simulink model "ModelG"  (Simulink 7.4)
settings: Solver=ode45  StartTime=0.0  StopTime=400  RelTol=1e-5
undefined symbols (not defined in the file): magnitude
settings Model: Creator=Lluís  LastModifiedBy=Lluís

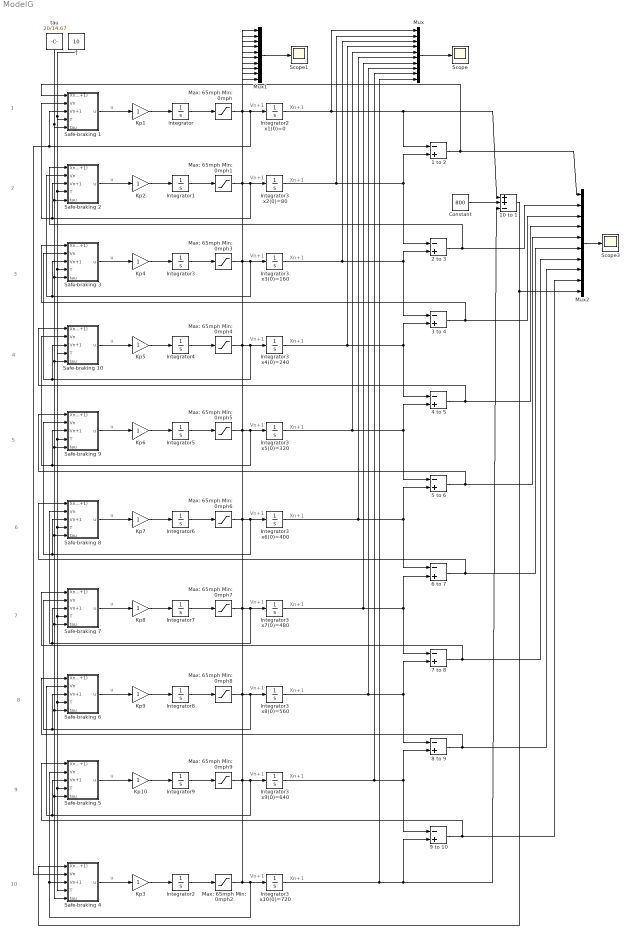
== system ModelG ==
  note: u
  note: Vn+1
  note: Xn+1
  note: u
  note: Vn+1
  note: Xn+1
  note: 1
  note: 2
  note: u
  note: Vn+1
  note: Xn+1
  note: 10
  note: u
  note: Vn+1
  note: Xn+1
  note: 3
  note: u
  note: Vn+1
  note: Xn+1
  note: 4
  note: u
  note: Vn+1
  note: Xn+1
  note: 5
  note: u
  note: Vn+1
  note: Xn+1
  note: 6
  note: u
  note: Vn+1
  note: Xn+1
  note: 7
  note: u
  note: Vn+1
  note: Xn+1
  note: 8
  note: u
  note: Vn+1
  note: Xn+1
  note: 9
  1 to 2 : Sum  Inputs=-+  OutDataType=fixdt(1, 16)  OutScaling=2^-10
  10 to 1 : Sum  Inputs=++-  OutDataType=fixdt(1, 16)  OutScaling=2^-10
  2 to 3 : Sum  Inputs=-+  OutDataType=fixdt(1, 16)  OutScaling=2^-10
  3 to 4 : Sum  Inputs=-+  OutDataType=fixdt(1, 16)  OutScaling=2^-10
  4 to 5 : Sum  Inputs=-+  OutDataType=fixdt(1, 16)  OutScaling=2^-10
  5 to 6 : Sum  Inputs=-+  OutDataType=fixdt(1, 16)  OutScaling=2^-10
  6 to 7 : Sum  Inputs=-+  OutDataType=fixdt(1, 16)  OutScaling=2^-10
  7 to 8 : Sum  Inputs=-+  OutDataType=fixdt(1, 16)  OutScaling=2^-10
  8 to 9 : Sum  Inputs=-+  OutDataType=fixdt(1, 16)  OutScaling=2^-10
  9 to 10 : Sum  Inputs=-+  OutDataType=fixdt(1, 16)  OutScaling=2^-10
  Constant : Constant  Value=800  OutDataType=fixdt(1, 16)  OutScaling=2^0
  Integrator : Integrator  InitialCondition=22
  Integrator{1..2,4,6,8} (5 alike) : Integrator  InitialCondition=66
  Integrator2 x1(0)=0 : Integrator
  Integrator3 : Integrator  InitialCondition=44
  Integrator3 x10(0)=720 : Integrator  InitialCondition=720
  Integrator3 x2(0)=80 : Integrator  InitialCondition=80
  Integrator3 x3(0)=160 : Integrator  InitialCondition=160
  Integrator3 x4(0)=240 : Integrator  InitialCondition=240
  Integrator3 x5(0)=320 : Integrator  InitialCondition=320
  Integrator3 x6(0)=400 : Integrator  InitialCondition=400
  Integrator3 x7(0)=480 : Integrator  InitialCondition=480
  Integrator3 x8(0)=560 : Integrator  InitialCondition=560
  Integrator3 x9(0)=640 : Integrator  InitialCondition=640
  Integrator5 : Integrator  InitialCondition=22
  Integrator7 : Integrator  InitialCondition=44
  Integrator9 : Integrator  InitialCondition=22
  Kp{1..10} (10 alike) : Gain  ParameterDataType=fixdt(1, 16)  ParameterScaling=2^0  OutDataType=fixdt(1, 16)  OutScaling=2^0
  Max: 65mph Min: 0mph{,1..9} (10 alike) : Saturate  UpperLimit=95.33  LowerLimit=0  OutDataType=fixdt(1, 16)  OutScaling=2^0
  Mux : Mux  Inputs=10
  Mux1 : Mux  Inputs=10
  Mux2 : Mux  Inputs=10
  Safe-braking 1 : Subsystem
  Safe-braking 10 : Subsystem
  Safe-braking 2 : Subsystem
  Safe-braking 3 : Subsystem
  Safe-braking 4 : Subsystem
  Safe-braking 5 : Subsystem
  Safe-braking 6 : Subsystem
  Safe-braking 7 : Subsystem
  Safe-braking 8 : Subsystem
  Safe-braking 9 : Subsystem
  Scope : Scope
      settings: SaveName=pos  DataFormat=Array
  Scope1 : Scope
      settings: SaveName=speed
  Scope3 : Scope
      settings: SaveName=ScopeData3
  T : Constant  Value=10  OutDataType=fixdt(1, 16)  OutScaling=2^0
  tau : Constant  Value=20/14.67  OutDataType=fixdt(1, 16)  OutScaling=2^0
  wires:
  1 to 2/1 -> Safe-braking 1/1(Xn-(Xn+1)), Mux2/1
  Max: 65mph Min: 0mph/1 -> Integrator2 x1(0)=0/1, Safe-braking 1/3(Vn+1), Safe-braking 4/2(Vn), Mux1/1
  Kp1/1 -> Integrator/1
  Safe-braking 1/1(u) -> Kp1/1
  Integrator/1 -> Max: 65mph Min: 0mph/1
  Integrator2 x1(0)=0/1 -> 1 to 2/1, 10 to 1/1, Mux/1
  Max: 65mph Min: 0mph1/1 -> Safe-braking 1/2(Vn), Safe-braking 2/3(Vn+1), Integrator3 x2(0)=80/1, Mux1/2
  Kp2/1 -> Integrator1/1
  Safe-braking 2/1(u) -> Kp2/1
  Integrator1/1 -> Max: 65mph Min: 0mph1/1
  Integrator3 x2(0)=80/1 -> 1 to 2/2, 2 to 3/1, Mux/2
  Max: 65mph Min: 0mph2/1 -> Integrator3 x10(0)=720/1, Safe-braking 4/3(Vn+1), Safe-braking 5/2(Vn), Mux1/10
  Kp3/1 -> Integrator2/1
  Safe-braking 4/1(u) -> Kp3/1
  Integrator2/1 -> Max: 65mph Min: 0mph2/1
  Integrator3 x10(0)=720/1 -> 10 to 1/3, 9 to 10/2, Mux/10
  2 to 3/1 -> Mux2/2, Safe-braking 2/1(Xn-(Xn+1))
  Constant/1 -> 10 to 1/2
  10 to 1/1 -> Mux2/10, Safe-braking 4/1(Xn-(Xn+1))
  Mux/1 -> Scope/1
  Mux1/1 -> Scope1/1
  Mux2/1 -> Scope3/1
  Max: 65mph Min: 0mph3/1 -> Integrator3 x3(0)=160/1, Safe-braking 2/2(Vn), Safe-braking 3/3(Vn+1), Mux1/3
  Kp4/1 -> Integrator3/1
  Safe-braking 3/1(u) -> Kp4/1
  Integrator3/1 -> Max: 65mph Min: 0mph3/1
  Integrator3 x3(0)=160/1 -> 2 to 3/2, 3 to 4/1, Mux/3
  3 to 4/1 -> Mux2/3, Safe-braking 3/1(Xn-(Xn+1))
  Max: 65mph Min: 0mph4/1 -> Integrator3 x4(0)=240/1, Safe-braking 3/2(Vn), Safe-braking 10/3(Vn+1), Mux1/4
  Kp5/1 -> Integrator4/1
  Safe-braking 10/1(u) -> Kp5/1
  Integrator4/1 -> Max: 65mph Min: 0mph4/1
  Integrator3 x4(0)=240/1 -> 3 to 4/2, 4 to 5/1, Mux/4
  4 to 5/1 -> Mux2/4, Safe-braking 10/1(Xn-(Xn+1))
  Max: 65mph Min: 0mph5/1 -> Integrator3 x5(0)=320/1, Safe-braking 9/3(Vn+1), Safe-braking 10/2(Vn), Mux1/5
  Kp6/1 -> Integrator5/1
  Safe-braking 9/1(u) -> Kp6/1
  Integrator5/1 -> Max: 65mph Min: 0mph5/1
  Integrator3 x5(0)=320/1 -> 4 to 5/2, 5 to 6/1, Mux/5
  5 to 6/1 -> Mux2/5, Safe-braking 9/1(Xn-(Xn+1))
  Max: 65mph Min: 0mph6/1 -> Integrator3 x6(0)=400/1, Safe-braking 8/3(Vn+1), Safe-braking 9/2(Vn), Mux1/6
  Kp7/1 -> Integrator6/1
  Safe-braking 8/1(u) -> Kp7/1
  Integrator6/1 -> Max: 65mph Min: 0mph6/1
  Integrator3 x6(0)=400/1 -> 5 to 6/2, 6 to 7/1, Mux/6
  6 to 7/1 -> Mux2/6, Safe-braking 8/1(Xn-(Xn+1))
  Max: 65mph Min: 0mph7/1 -> Integrator3 x7(0)=480/1, Safe-braking 7/3(Vn+1), Safe-braking 8/2(Vn), Mux1/7
  Kp8/1 -> Integrator7/1
  Safe-braking 7/1(u) -> Kp8/1
  Integrator7/1 -> Max: 65mph Min: 0mph7/1
  Integrator3 x7(0)=480/1 -> 6 to 7/2, 7 to 8/1, Mux/7
  7 to 8/1 -> Mux2/7, Safe-braking 7/1(Xn-(Xn+1))
  Max: 65mph Min: 0mph8/1 -> Integrator3 x8(0)=560/1, Safe-braking 6/3(Vn+1), Safe-braking 7/2(Vn), Mux1/8
  Kp9/1 -> Integrator8/1
  Safe-braking 6/1(u) -> Kp9/1
  Integrator8/1 -> Max: 65mph Min: 0mph8/1
  Integrator3 x8(0)=560/1 -> 7 to 8/2, 8 to 9/1, Mux/8
  8 to 9/1 -> Mux2/8, Safe-braking 6/1(Xn-(Xn+1))
  Max: 65mph Min: 0mph9/1 -> Integrator3 x9(0)=640/1, Safe-braking 5/3(Vn+1), Safe-braking 6/2(Vn), Mux1/9
  Kp10/1 -> Integrator9/1
  Safe-braking 5/1(u) -> Kp10/1
  Integrator9/1 -> Max: 65mph Min: 0mph9/1
  Integrator3 x9(0)=640/1 -> 8 to 9/2, 9 to 10/1, Mux/9
  9 to 10/1 -> Mux2/9, Safe-braking 5/1(Xn-(Xn+1))
  T/1 -> Safe-braking 2/4(T), Safe-braking 3/4(T), Safe-braking 9/4(T), Safe-braking 8/4(T), Safe-braking 7/4(T), Safe-braking 6/4(T), Safe-braking 5/4(T), Safe-braking 4/4(T), Safe-braking 10/4(T), Safe-braking 1/4(T)
  tau/1 -> Safe-braking 2/5(tau), Safe-braking 3/5(tau), Safe-braking 10/5(tau), Safe-braking 9/5(tau), Safe-braking 8/5(tau), Safe-braking 7/5(tau), Safe-braking 6/5(tau), Safe-braking 5/5(tau), Safe-braking 4/5(tau), Safe-braking 1/5(tau)

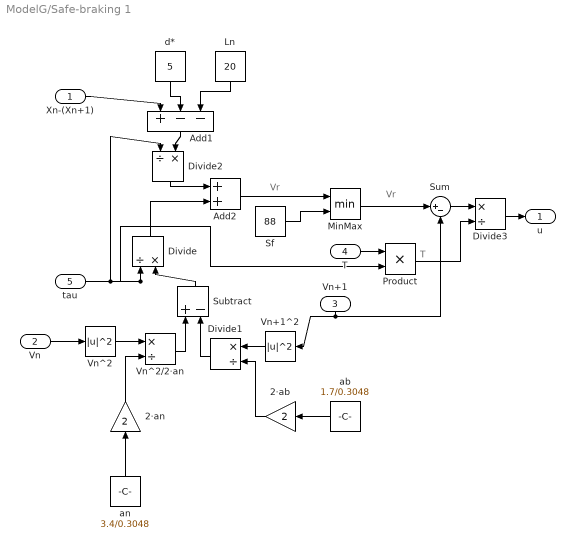
== system ModelG/Safe-braking 1 ==
  note: Vr
  note: Vr
  note: T
  Xn-(Xn+1) : Inport
  Vn : Inport  Port=2
  Vn+1 : Inport  Port=3
  T : Inport  Port=4  OutDataType=fixdt(1, 16)  OutScaling=2^0
  tau : Inport  Port=5  OutDataType=fixdt(1, 16)  OutScaling=2^0
  2·ab : Gain  Gain=2  ParameterDataType=fixdt(1, 16)  ParameterScaling=2^0  OutDataType=fixdt(1, 16)  OutScaling=2^0
  2·an : Gain  Gain=2  ParameterDataType=fixdt(1, 16)  ParameterScaling=2^0  OutDataType=fixdt(1, 16)  OutScaling=2^0
  Add1 : Sum  Inputs=+--  OutDataType=fixdt(1, 16)  OutScaling=2^-10
  Add2 : Sum  OutDataType=fixdt(1, 16)  OutScaling=2^-10
  Divide : Product  Inputs=/*  OutDataType=fixdt(1, 16)  OutScaling=2^-10
  Divide1 : Product  Inputs=*/  OutDataType=fixdt(1, 16)  OutScaling=2^-10
  Divide2 : Product  Inputs=/*  OutDataType=fixdt(1, 16)  OutScaling=2^-10
  Divide3 : Product  Inputs=*/  OutDataType=fixdt(1, 16)  OutScaling=2^-10
  Ln : Constant  Value=20  OutDataType=fixdt(1, 16)  OutScaling=2^0
  MinMax : MinMax  Inputs=2  OutDataType=fixdt(1, 16)  OutScaling=2^0
  Product : Product  OutDataType=fixdt(1, 16)  OutScaling=2^0  RndMeth=Zero
  Sf : Constant  Value=88  OutDataType=fixdt(1, 16)  OutScaling=2^0
  Subtract : Sum  Inputs=+-  OutDataType=fixdt(1, 16)  OutScaling=2^-10
  Sum : Sum  Inputs=|+-  OutDataType=fixdt(1, 16)  OutScaling=2^0
  Vn+1^2 : Math  Operator=magnitude^2  OutDataType=fixdt(1, 16)  OutScaling=2^0  SaturateOnIntegerOverflow=on
  Vn^2 : Math  Operator=magnitude^2  OutDataType=fixdt(1, 16)  OutScaling=2^0  SaturateOnIntegerOverflow=on
  Vn^2/2·an : Product  Inputs=*/  OutDataType=fixdt(1, 16)  OutScaling=2^-10
  ab : Constant  Value=1.7/0.3048  OutDataType=fixdt(1, 16)  OutScaling=2^0
  an : Constant  Value=3.4/0.3048  OutDataType=fixdt(1, 16)  OutScaling=2^0
  d* : Constant  Value=5  OutDataType=fixdt(1, 16)  OutScaling=2^0
  u : Outport
  wires:
  ab/1 -> 2·ab/1
  Vn^2/1 -> Vn^2/2·an/1
  2·an/1 -> Vn^2/2·an/2
  Vn+1^2/1 -> Divide1/1
  2·ab/1 -> Divide1/2
  Vn^2/2·an/1 -> Subtract/1
  Divide1/1 -> Subtract/2
  Subtract/1 -> Divide/2
  tau/1 -> Divide2/1, Divide/1, Product/2
  d*/1 -> Add1/2
  Ln/1 -> Add1/3
  Add1/1 -> Divide2/2
  Divide2/1 -> Add2/1
  Divide/1 -> Add2/2
  Xn-(Xn+1)/1 -> Add1/1
  Vn/1 -> Vn^2/1
  Vn+1/1 -> Vn+1^2/1, Sum/2
  an/1 -> 2·an/1
  Add2/1 -> MinMax/1
  Sf/1 -> MinMax/2
  MinMax/1 -> Sum/1
  Sum/1 -> Divide3/1
  Product/1 -> Divide3/2
  Divide3/1 -> u/1
  T/1 -> Product/1

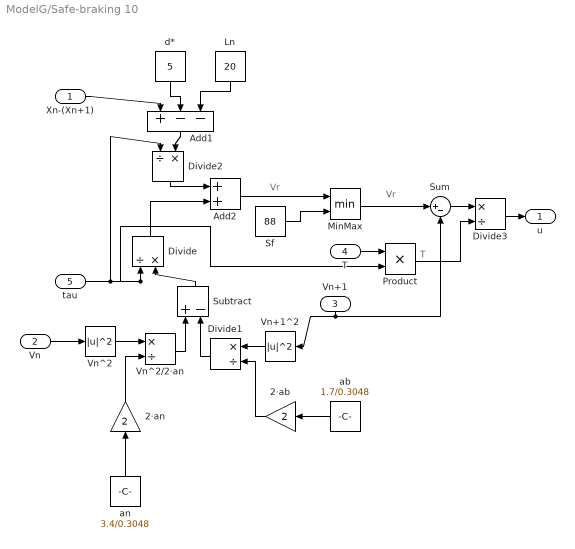
== system ModelG/Safe-braking 10 ==
  note: Vr
  note: Vr
  note: T
  Xn-(Xn+1) : Inport
  Vn : Inport  Port=2
  Vn+1 : Inport  Port=3
  T : Inport  Port=4  OutDataType=fixdt(1, 16)  OutScaling=2^0
  tau : Inport  Port=5  OutDataType=fixdt(1, 16)  OutScaling=2^0
  2·ab : Gain  Gain=2  ParameterDataType=fixdt(1, 16)  ParameterScaling=2^0  OutDataType=fixdt(1, 16)  OutScaling=2^0
  2·an : Gain  Gain=2  ParameterDataType=fixdt(1, 16)  ParameterScaling=2^0  OutDataType=fixdt(1, 16)  OutScaling=2^0
  Add1 : Sum  Inputs=+--  OutDataType=fixdt(1, 16)  OutScaling=2^-10
  Add2 : Sum  OutDataType=fixdt(1, 16)  OutScaling=2^-10
  Divide : Product  Inputs=/*  OutDataType=fixdt(1, 16)  OutScaling=2^-10
  Divide1 : Product  Inputs=*/  OutDataType=fixdt(1, 16)  OutScaling=2^-10
  Divide2 : Product  Inputs=/*  OutDataType=fixdt(1, 16)  OutScaling=2^-10
  Divide3 : Product  Inputs=*/  OutDataType=fixdt(1, 16)  OutScaling=2^-10
  Ln : Constant  Value=20  OutDataType=fixdt(1, 16)  OutScaling=2^0
  MinMax : MinMax  Inputs=2  OutDataType=fixdt(1, 16)  OutScaling=2^0
  Product : Product  OutDataType=fixdt(1, 16)  OutScaling=2^0  RndMeth=Zero
  Sf : Constant  Value=88  OutDataType=fixdt(1, 16)  OutScaling=2^0
  Subtract : Sum  Inputs=+-  OutDataType=fixdt(1, 16)  OutScaling=2^-10
  Sum : Sum  Inputs=|+-  OutDataType=fixdt(1, 16)  OutScaling=2^0
  Vn+1^2 : Math  Operator=magnitude^2  OutDataType=fixdt(1, 16)  OutScaling=2^0  SaturateOnIntegerOverflow=on
  Vn^2 : Math  Operator=magnitude^2  OutDataType=fixdt(1, 16)  OutScaling=2^0  SaturateOnIntegerOverflow=on
  Vn^2/2·an : Product  Inputs=*/  OutDataType=fixdt(1, 16)  OutScaling=2^-10
  ab : Constant  Value=1.7/0.3048  OutDataType=fixdt(1, 16)  OutScaling=2^0
  an : Constant  Value=3.4/0.3048  OutDataType=fixdt(1, 16)  OutScaling=2^0
  d* : Constant  Value=5  OutDataType=fixdt(1, 16)  OutScaling=2^0
  u : Outport
  wires:
  ab/1 -> 2·ab/1
  Vn^2/1 -> Vn^2/2·an/1
  2·an/1 -> Vn^2/2·an/2
  Vn+1^2/1 -> Divide1/1
  2·ab/1 -> Divide1/2
  Vn^2/2·an/1 -> Subtract/1
  Divide1/1 -> Subtract/2
  Subtract/1 -> Divide/2
  tau/1 -> Divide2/1, Divide/1, Product/2
  d*/1 -> Add1/2
  Ln/1 -> Add1/3
  Add1/1 -> Divide2/2
  Divide2/1 -> Add2/1
  Divide/1 -> Add2/2
  Xn-(Xn+1)/1 -> Add1/1
  Vn/1 -> Vn^2/1
  Vn+1/1 -> Vn+1^2/1, Sum/2
  an/1 -> 2·an/1
  Add2/1 -> MinMax/1
  Sf/1 -> MinMax/2
  MinMax/1 -> Sum/1
  Sum/1 -> Divide3/1
  Product/1 -> Divide3/2
  Divide3/1 -> u/1
  T/1 -> Product/1

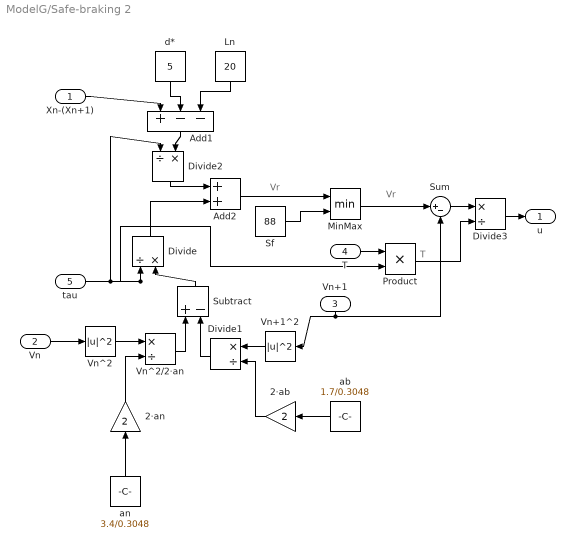
== system ModelG/Safe-braking 2 ==
  note: Vr
  note: Vr
  note: T
  Xn-(Xn+1) : Inport
  Vn : Inport  Port=2
  Vn+1 : Inport  Port=3
  T : Inport  Port=4  OutDataType=fixdt(1, 16)  OutScaling=2^0
  tau : Inport  Port=5  OutDataType=fixdt(1, 16)  OutScaling=2^0
  2·ab : Gain  Gain=2  ParameterDataType=fixdt(1, 16)  ParameterScaling=2^0  OutDataType=fixdt(1, 16)  OutScaling=2^0
  2·an : Gain  Gain=2  ParameterDataType=fixdt(1, 16)  ParameterScaling=2^0  OutDataType=fixdt(1, 16)  OutScaling=2^0
  Add1 : Sum  Inputs=+--  OutDataType=fixdt(1, 16)  OutScaling=2^-10
  Add2 : Sum  OutDataType=fixdt(1, 16)  OutScaling=2^-10
  Divide : Product  Inputs=/*  OutDataType=fixdt(1, 16)  OutScaling=2^-10
  Divide1 : Product  Inputs=*/  OutDataType=fixdt(1, 16)  OutScaling=2^-10
  Divide2 : Product  Inputs=/*  OutDataType=fixdt(1, 16)  OutScaling=2^-10
  Divide3 : Product  Inputs=*/  OutDataType=fixdt(1, 16)  OutScaling=2^-10
  Ln : Constant  Value=20  OutDataType=fixdt(1, 16)  OutScaling=2^0
  MinMax : MinMax  Inputs=2  OutDataType=fixdt(1, 16)  OutScaling=2^0
  Product : Product  OutDataType=fixdt(1, 16)  OutScaling=2^0  RndMeth=Zero
  Sf : Constant  Value=88  OutDataType=fixdt(1, 16)  OutScaling=2^0
  Subtract : Sum  Inputs=+-  OutDataType=fixdt(1, 16)  OutScaling=2^-10
  Sum : Sum  Inputs=|+-  OutDataType=fixdt(1, 16)  OutScaling=2^0
  Vn+1^2 : Math  Operator=magnitude^2  OutDataType=fixdt(1, 16)  OutScaling=2^0  SaturateOnIntegerOverflow=on
  Vn^2 : Math  Operator=magnitude^2  OutDataType=fixdt(1, 16)  OutScaling=2^0  SaturateOnIntegerOverflow=on
  Vn^2/2·an : Product  Inputs=*/  OutDataType=fixdt(1, 16)  OutScaling=2^-10
  ab : Constant  Value=1.7/0.3048  OutDataType=fixdt(1, 16)  OutScaling=2^0
  an : Constant  Value=3.4/0.3048  OutDataType=fixdt(1, 16)  OutScaling=2^0
  d* : Constant  Value=5  OutDataType=fixdt(1, 16)  OutScaling=2^0
  u : Outport
  wires:
  ab/1 -> 2·ab/1
  Vn^2/1 -> Vn^2/2·an/1
  2·an/1 -> Vn^2/2·an/2
  Vn+1^2/1 -> Divide1/1
  2·ab/1 -> Divide1/2
  Vn^2/2·an/1 -> Subtract/1
  Divide1/1 -> Subtract/2
  Subtract/1 -> Divide/2
  tau/1 -> Divide2/1, Divide/1, Product/2
  d*/1 -> Add1/2
  Ln/1 -> Add1/3
  Add1/1 -> Divide2/2
  Divide2/1 -> Add2/1
  Divide/1 -> Add2/2
  Xn-(Xn+1)/1 -> Add1/1
  Vn/1 -> Vn^2/1
  Vn+1/1 -> Vn+1^2/1, Sum/2
  an/1 -> 2·an/1
  Add2/1 -> MinMax/1
  Sf/1 -> MinMax/2
  MinMax/1 -> Sum/1
  Sum/1 -> Divide3/1
  Product/1 -> Divide3/2
  Divide3/1 -> u/1
  T/1 -> Product/1

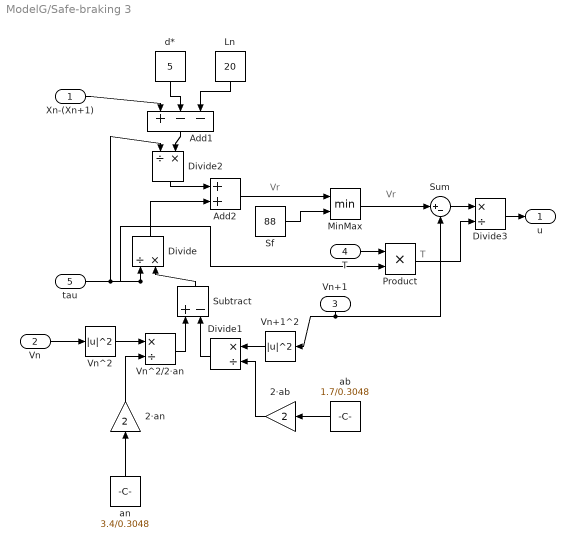
== system ModelG/Safe-braking 3 ==
  note: Vr
  note: Vr
  note: T
  Xn-(Xn+1) : Inport
  Vn : Inport  Port=2
  Vn+1 : Inport  Port=3
  T : Inport  Port=4  OutDataType=fixdt(1, 16)  OutScaling=2^0
  tau : Inport  Port=5  OutDataType=fixdt(1, 16)  OutScaling=2^0
  2·ab : Gain  Gain=2  ParameterDataType=fixdt(1, 16)  ParameterScaling=2^0  OutDataType=fixdt(1, 16)  OutScaling=2^0
  2·an : Gain  Gain=2  ParameterDataType=fixdt(1, 16)  ParameterScaling=2^0  OutDataType=fixdt(1, 16)  OutScaling=2^0
  Add1 : Sum  Inputs=+--  OutDataType=fixdt(1, 16)  OutScaling=2^-10
  Add2 : Sum  OutDataType=fixdt(1, 16)  OutScaling=2^-10
  Divide : Product  Inputs=/*  OutDataType=fixdt(1, 16)  OutScaling=2^-10
  Divide1 : Product  Inputs=*/  OutDataType=fixdt(1, 16)  OutScaling=2^-10
  Divide2 : Product  Inputs=/*  OutDataType=fixdt(1, 16)  OutScaling=2^-10
  Divide3 : Product  Inputs=*/  OutDataType=fixdt(1, 16)  OutScaling=2^-10
  Ln : Constant  Value=20  OutDataType=fixdt(1, 16)  OutScaling=2^0
  MinMax : MinMax  Inputs=2  OutDataType=fixdt(1, 16)  OutScaling=2^0
  Product : Product  OutDataType=fixdt(1, 16)  OutScaling=2^0  RndMeth=Zero
  Sf : Constant  Value=88  OutDataType=fixdt(1, 16)  OutScaling=2^0
  Subtract : Sum  Inputs=+-  OutDataType=fixdt(1, 16)  OutScaling=2^-10
  Sum : Sum  Inputs=|+-  OutDataType=fixdt(1, 16)  OutScaling=2^0
  Vn+1^2 : Math  Operator=magnitude^2  OutDataType=fixdt(1, 16)  OutScaling=2^0  SaturateOnIntegerOverflow=on
  Vn^2 : Math  Operator=magnitude^2  OutDataType=fixdt(1, 16)  OutScaling=2^0  SaturateOnIntegerOverflow=on
  Vn^2/2·an : Product  Inputs=*/  OutDataType=fixdt(1, 16)  OutScaling=2^-10
  ab : Constant  Value=1.7/0.3048  OutDataType=fixdt(1, 16)  OutScaling=2^0
  an : Constant  Value=3.4/0.3048  OutDataType=fixdt(1, 16)  OutScaling=2^0
  d* : Constant  Value=5  OutDataType=fixdt(1, 16)  OutScaling=2^0
  u : Outport
  wires:
  ab/1 -> 2·ab/1
  Vn^2/1 -> Vn^2/2·an/1
  2·an/1 -> Vn^2/2·an/2
  Vn+1^2/1 -> Divide1/1
  2·ab/1 -> Divide1/2
  Vn^2/2·an/1 -> Subtract/1
  Divide1/1 -> Subtract/2
  Subtract/1 -> Divide/2
  tau/1 -> Divide2/1, Divide/1, Product/2
  d*/1 -> Add1/2
  Ln/1 -> Add1/3
  Add1/1 -> Divide2/2
  Divide2/1 -> Add2/1
  Divide/1 -> Add2/2
  Xn-(Xn+1)/1 -> Add1/1
  Vn/1 -> Vn^2/1
  Vn+1/1 -> Vn+1^2/1, Sum/2
  an/1 -> 2·an/1
  Add2/1 -> MinMax/1
  Sf/1 -> MinMax/2
  MinMax/1 -> Sum/1
  Sum/1 -> Divide3/1
  Product/1 -> Divide3/2
  Divide3/1 -> u/1
  T/1 -> Product/1

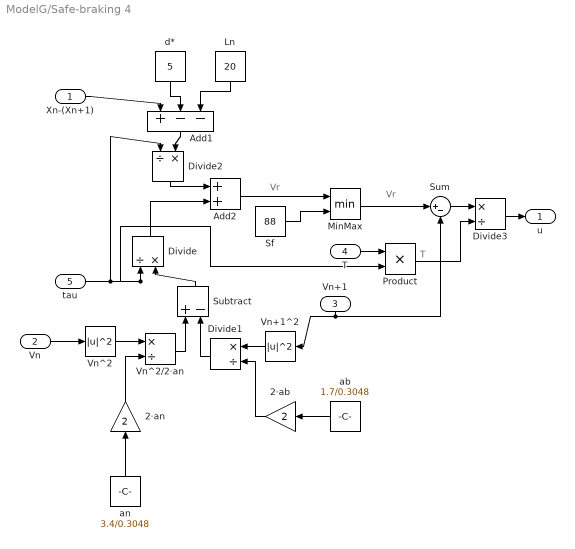
== system ModelG/Safe-braking 4 ==
  note: Vr
  note: Vr
  note: T
  Xn-(Xn+1) : Inport
  Vn : Inport  Port=2
  Vn+1 : Inport  Port=3
  T : Inport  Port=4  OutDataType=fixdt(1, 16)  OutScaling=2^0
  tau : Inport  Port=5  OutDataType=fixdt(1, 16)  OutScaling=2^0
  2·ab : Gain  Gain=2  ParameterDataType=fixdt(1, 16)  ParameterScaling=2^0  OutDataType=fixdt(1, 16)  OutScaling=2^0
  2·an : Gain  Gain=2  ParameterDataType=fixdt(1, 16)  ParameterScaling=2^0  OutDataType=fixdt(1, 16)  OutScaling=2^0
  Add1 : Sum  Inputs=+--  OutDataType=fixdt(1, 16)  OutScaling=2^-10
  Add2 : Sum  OutDataType=fixdt(1, 16)  OutScaling=2^-10
  Divide : Product  Inputs=/*  OutDataType=fixdt(1, 16)  OutScaling=2^-10
  Divide1 : Product  Inputs=*/  OutDataType=fixdt(1, 16)  OutScaling=2^-10
  Divide2 : Product  Inputs=/*  OutDataType=fixdt(1, 16)  OutScaling=2^-10
  Divide3 : Product  Inputs=*/  OutDataType=fixdt(1, 16)  OutScaling=2^-10
  Ln : Constant  Value=20  OutDataType=fixdt(1, 16)  OutScaling=2^0
  MinMax : MinMax  Inputs=2  OutDataType=fixdt(1, 16)  OutScaling=2^0
  Product : Product  OutDataType=fixdt(1, 16)  OutScaling=2^0  RndMeth=Zero
  Sf : Constant  Value=88  OutDataType=fixdt(1, 16)  OutScaling=2^0
  Subtract : Sum  Inputs=+-  OutDataType=fixdt(1, 16)  OutScaling=2^-10
  Sum : Sum  Inputs=|+-  OutDataType=fixdt(1, 16)  OutScaling=2^0
  Vn+1^2 : Math  Operator=magnitude^2  OutDataType=fixdt(1, 16)  OutScaling=2^0  SaturateOnIntegerOverflow=on
  Vn^2 : Math  Operator=magnitude^2  OutDataType=fixdt(1, 16)  OutScaling=2^0  SaturateOnIntegerOverflow=on
  Vn^2/2·an : Product  Inputs=*/  OutDataType=fixdt(1, 16)  OutScaling=2^-10
  ab : Constant  Value=1.7/0.3048  OutDataType=fixdt(1, 16)  OutScaling=2^0
  an : Constant  Value=3.4/0.3048  OutDataType=fixdt(1, 16)  OutScaling=2^0
  d* : Constant  Value=5  OutDataType=fixdt(1, 16)  OutScaling=2^0
  u : Outport
  wires:
  ab/1 -> 2·ab/1
  Vn^2/1 -> Vn^2/2·an/1
  2·an/1 -> Vn^2/2·an/2
  Vn+1^2/1 -> Divide1/1
  2·ab/1 -> Divide1/2
  Vn^2/2·an/1 -> Subtract/1
  Divide1/1 -> Subtract/2
  Subtract/1 -> Divide/2
  tau/1 -> Divide2/1, Divide/1, Product/2
  d*/1 -> Add1/2
  Ln/1 -> Add1/3
  Add1/1 -> Divide2/2
  Divide2/1 -> Add2/1
  Divide/1 -> Add2/2
  Xn-(Xn+1)/1 -> Add1/1
  Vn/1 -> Vn^2/1
  Vn+1/1 -> Vn+1^2/1, Sum/2
  an/1 -> 2·an/1
  Add2/1 -> MinMax/1
  Sf/1 -> MinMax/2
  MinMax/1 -> Sum/1
  Sum/1 -> Divide3/1
  Product/1 -> Divide3/2
  Divide3/1 -> u/1
  T/1 -> Product/1

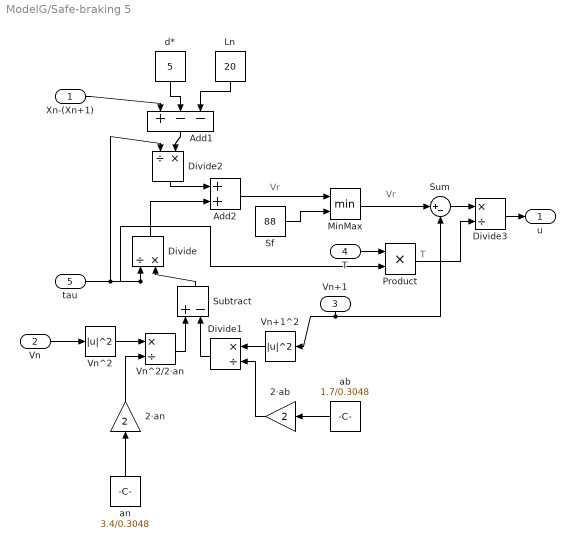
== system ModelG/Safe-braking 5 ==
  note: Vr
  note: Vr
  note: T
  Xn-(Xn+1) : Inport
  Vn : Inport  Port=2
  Vn+1 : Inport  Port=3
  T : Inport  Port=4  OutDataType=fixdt(1, 16)  OutScaling=2^0
  tau : Inport  Port=5  OutDataType=fixdt(1, 16)  OutScaling=2^0
  2·ab : Gain  Gain=2  ParameterDataType=fixdt(1, 16)  ParameterScaling=2^0  OutDataType=fixdt(1, 16)  OutScaling=2^0
  2·an : Gain  Gain=2  ParameterDataType=fixdt(1, 16)  ParameterScaling=2^0  OutDataType=fixdt(1, 16)  OutScaling=2^0
  Add1 : Sum  Inputs=+--  OutDataType=fixdt(1, 16)  OutScaling=2^-10
  Add2 : Sum  OutDataType=fixdt(1, 16)  OutScaling=2^-10
  Divide : Product  Inputs=/*  OutDataType=fixdt(1, 16)  OutScaling=2^-10
  Divide1 : Product  Inputs=*/  OutDataType=fixdt(1, 16)  OutScaling=2^-10
  Divide2 : Product  Inputs=/*  OutDataType=fixdt(1, 16)  OutScaling=2^-10
  Divide3 : Product  Inputs=*/  OutDataType=fixdt(1, 16)  OutScaling=2^-10
  Ln : Constant  Value=20  OutDataType=fixdt(1, 16)  OutScaling=2^0
  MinMax : MinMax  Inputs=2  OutDataType=fixdt(1, 16)  OutScaling=2^0
  Product : Product  OutDataType=fixdt(1, 16)  OutScaling=2^0  RndMeth=Zero
  Sf : Constant  Value=88  OutDataType=fixdt(1, 16)  OutScaling=2^0
  Subtract : Sum  Inputs=+-  OutDataType=fixdt(1, 16)  OutScaling=2^-10
  Sum : Sum  Inputs=|+-  OutDataType=fixdt(1, 16)  OutScaling=2^0
  Vn+1^2 : Math  Operator=magnitude^2  OutDataType=fixdt(1, 16)  OutScaling=2^0  SaturateOnIntegerOverflow=on
  Vn^2 : Math  Operator=magnitude^2  OutDataType=fixdt(1, 16)  OutScaling=2^0  SaturateOnIntegerOverflow=on
  Vn^2/2·an : Product  Inputs=*/  OutDataType=fixdt(1, 16)  OutScaling=2^-10
  ab : Constant  Value=1.7/0.3048  OutDataType=fixdt(1, 16)  OutScaling=2^0
  an : Constant  Value=3.4/0.3048  OutDataType=fixdt(1, 16)  OutScaling=2^0
  d* : Constant  Value=5  OutDataType=fixdt(1, 16)  OutScaling=2^0
  u : Outport
  wires:
  ab/1 -> 2·ab/1
  Vn^2/1 -> Vn^2/2·an/1
  2·an/1 -> Vn^2/2·an/2
  Vn+1^2/1 -> Divide1/1
  2·ab/1 -> Divide1/2
  Vn^2/2·an/1 -> Subtract/1
  Divide1/1 -> Subtract/2
  Subtract/1 -> Divide/2
  tau/1 -> Divide2/1, Divide/1, Product/2
  d*/1 -> Add1/2
  Ln/1 -> Add1/3
  Add1/1 -> Divide2/2
  Divide2/1 -> Add2/1
  Divide/1 -> Add2/2
  Xn-(Xn+1)/1 -> Add1/1
  Vn/1 -> Vn^2/1
  Vn+1/1 -> Vn+1^2/1, Sum/2
  an/1 -> 2·an/1
  Add2/1 -> MinMax/1
  Sf/1 -> MinMax/2
  MinMax/1 -> Sum/1
  Sum/1 -> Divide3/1
  Product/1 -> Divide3/2
  Divide3/1 -> u/1
  T/1 -> Product/1

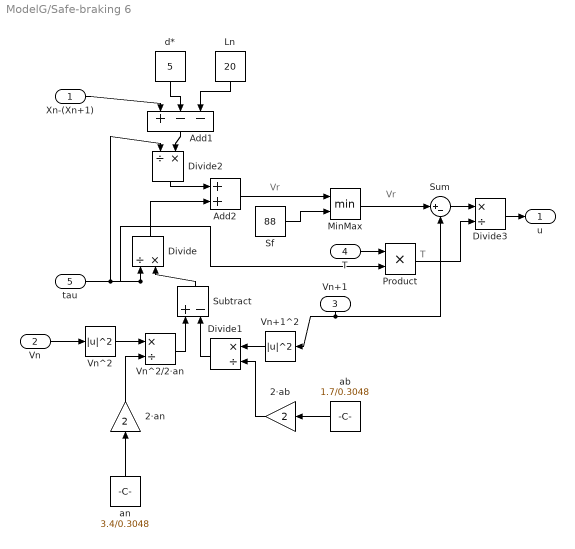
== system ModelG/Safe-braking 6 ==
  note: Vr
  note: Vr
  note: T
  Xn-(Xn+1) : Inport
  Vn : Inport  Port=2
  Vn+1 : Inport  Port=3
  T : Inport  Port=4  OutDataType=fixdt(1, 16)  OutScaling=2^0
  tau : Inport  Port=5  OutDataType=fixdt(1, 16)  OutScaling=2^0
  2·ab : Gain  Gain=2  ParameterDataType=fixdt(1, 16)  ParameterScaling=2^0  OutDataType=fixdt(1, 16)  OutScaling=2^0
  2·an : Gain  Gain=2  ParameterDataType=fixdt(1, 16)  ParameterScaling=2^0  OutDataType=fixdt(1, 16)  OutScaling=2^0
  Add1 : Sum  Inputs=+--  OutDataType=fixdt(1, 16)  OutScaling=2^-10
  Add2 : Sum  OutDataType=fixdt(1, 16)  OutScaling=2^-10
  Divide : Product  Inputs=/*  OutDataType=fixdt(1, 16)  OutScaling=2^-10
  Divide1 : Product  Inputs=*/  OutDataType=fixdt(1, 16)  OutScaling=2^-10
  Divide2 : Product  Inputs=/*  OutDataType=fixdt(1, 16)  OutScaling=2^-10
  Divide3 : Product  Inputs=*/  OutDataType=fixdt(1, 16)  OutScaling=2^-10
  Ln : Constant  Value=20  OutDataType=fixdt(1, 16)  OutScaling=2^0
  MinMax : MinMax  Inputs=2  OutDataType=fixdt(1, 16)  OutScaling=2^0
  Product : Product  OutDataType=fixdt(1, 16)  OutScaling=2^0  RndMeth=Zero
  Sf : Constant  Value=88  OutDataType=fixdt(1, 16)  OutScaling=2^0
  Subtract : Sum  Inputs=+-  OutDataType=fixdt(1, 16)  OutScaling=2^-10
  Sum : Sum  Inputs=|+-  OutDataType=fixdt(1, 16)  OutScaling=2^0
  Vn+1^2 : Math  Operator=magnitude^2  OutDataType=fixdt(1, 16)  OutScaling=2^0  SaturateOnIntegerOverflow=on
  Vn^2 : Math  Operator=magnitude^2  OutDataType=fixdt(1, 16)  OutScaling=2^0  SaturateOnIntegerOverflow=on
  Vn^2/2·an : Product  Inputs=*/  OutDataType=fixdt(1, 16)  OutScaling=2^-10
  ab : Constant  Value=1.7/0.3048  OutDataType=fixdt(1, 16)  OutScaling=2^0
  an : Constant  Value=3.4/0.3048  OutDataType=fixdt(1, 16)  OutScaling=2^0
  d* : Constant  Value=5  OutDataType=fixdt(1, 16)  OutScaling=2^0
  u : Outport
  wires:
  ab/1 -> 2·ab/1
  Vn^2/1 -> Vn^2/2·an/1
  2·an/1 -> Vn^2/2·an/2
  Vn+1^2/1 -> Divide1/1
  2·ab/1 -> Divide1/2
  Vn^2/2·an/1 -> Subtract/1
  Divide1/1 -> Subtract/2
  Subtract/1 -> Divide/2
  tau/1 -> Divide2/1, Divide/1, Product/2
  d*/1 -> Add1/2
  Ln/1 -> Add1/3
  Add1/1 -> Divide2/2
  Divide2/1 -> Add2/1
  Divide/1 -> Add2/2
  Xn-(Xn+1)/1 -> Add1/1
  Vn/1 -> Vn^2/1
  Vn+1/1 -> Vn+1^2/1, Sum/2
  an/1 -> 2·an/1
  Add2/1 -> MinMax/1
  Sf/1 -> MinMax/2
  MinMax/1 -> Sum/1
  Sum/1 -> Divide3/1
  Product/1 -> Divide3/2
  Divide3/1 -> u/1
  T/1 -> Product/1

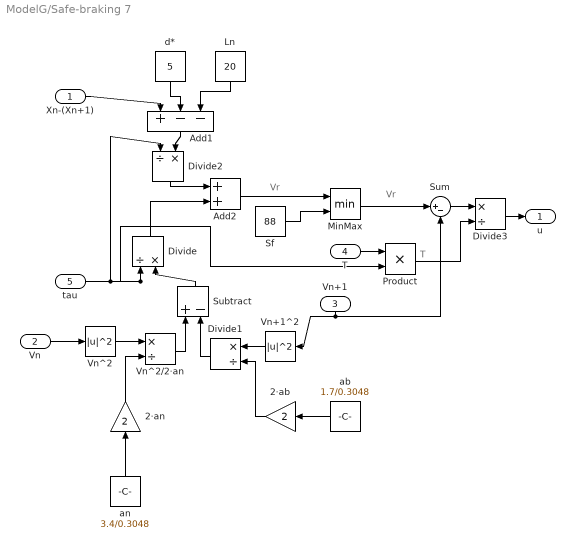
== system ModelG/Safe-braking 7 ==
  note: Vr
  note: Vr
  note: T
  Xn-(Xn+1) : Inport
  Vn : Inport  Port=2
  Vn+1 : Inport  Port=3
  T : Inport  Port=4  OutDataType=fixdt(1, 16)  OutScaling=2^0
  tau : Inport  Port=5  OutDataType=fixdt(1, 16)  OutScaling=2^0
  2·ab : Gain  Gain=2  ParameterDataType=fixdt(1, 16)  ParameterScaling=2^0  OutDataType=fixdt(1, 16)  OutScaling=2^0
  2·an : Gain  Gain=2  ParameterDataType=fixdt(1, 16)  ParameterScaling=2^0  OutDataType=fixdt(1, 16)  OutScaling=2^0
  Add1 : Sum  Inputs=+--  OutDataType=fixdt(1, 16)  OutScaling=2^-10
  Add2 : Sum  OutDataType=fixdt(1, 16)  OutScaling=2^-10
  Divide : Product  Inputs=/*  OutDataType=fixdt(1, 16)  OutScaling=2^-10
  Divide1 : Product  Inputs=*/  OutDataType=fixdt(1, 16)  OutScaling=2^-10
  Divide2 : Product  Inputs=/*  OutDataType=fixdt(1, 16)  OutScaling=2^-10
  Divide3 : Product  Inputs=*/  OutDataType=fixdt(1, 16)  OutScaling=2^-10
  Ln : Constant  Value=20  OutDataType=fixdt(1, 16)  OutScaling=2^0
  MinMax : MinMax  Inputs=2  OutDataType=fixdt(1, 16)  OutScaling=2^0
  Product : Product  OutDataType=fixdt(1, 16)  OutScaling=2^0  RndMeth=Zero
  Sf : Constant  Value=88  OutDataType=fixdt(1, 16)  OutScaling=2^0
  Subtract : Sum  Inputs=+-  OutDataType=fixdt(1, 16)  OutScaling=2^-10
  Sum : Sum  Inputs=|+-  OutDataType=fixdt(1, 16)  OutScaling=2^0
  Vn+1^2 : Math  Operator=magnitude^2  OutDataType=fixdt(1, 16)  OutScaling=2^0  SaturateOnIntegerOverflow=on
  Vn^2 : Math  Operator=magnitude^2  OutDataType=fixdt(1, 16)  OutScaling=2^0  SaturateOnIntegerOverflow=on
  Vn^2/2·an : Product  Inputs=*/  OutDataType=fixdt(1, 16)  OutScaling=2^-10
  ab : Constant  Value=1.7/0.3048  OutDataType=fixdt(1, 16)  OutScaling=2^0
  an : Constant  Value=3.4/0.3048  OutDataType=fixdt(1, 16)  OutScaling=2^0
  d* : Constant  Value=5  OutDataType=fixdt(1, 16)  OutScaling=2^0
  u : Outport
  wires:
  ab/1 -> 2·ab/1
  Vn^2/1 -> Vn^2/2·an/1
  2·an/1 -> Vn^2/2·an/2
  Vn+1^2/1 -> Divide1/1
  2·ab/1 -> Divide1/2
  Vn^2/2·an/1 -> Subtract/1
  Divide1/1 -> Subtract/2
  Subtract/1 -> Divide/2
  tau/1 -> Divide2/1, Divide/1, Product/2
  d*/1 -> Add1/2
  Ln/1 -> Add1/3
  Add1/1 -> Divide2/2
  Divide2/1 -> Add2/1
  Divide/1 -> Add2/2
  Xn-(Xn+1)/1 -> Add1/1
  Vn/1 -> Vn^2/1
  Vn+1/1 -> Vn+1^2/1, Sum/2
  an/1 -> 2·an/1
  Add2/1 -> MinMax/1
  Sf/1 -> MinMax/2
  MinMax/1 -> Sum/1
  Sum/1 -> Divide3/1
  Product/1 -> Divide3/2
  Divide3/1 -> u/1
  T/1 -> Product/1

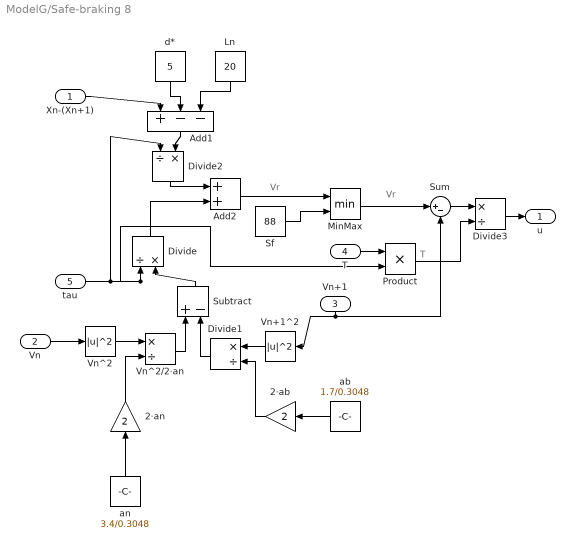
== system ModelG/Safe-braking 8 ==
  note: Vr
  note: Vr
  note: T
  Xn-(Xn+1) : Inport
  Vn : Inport  Port=2
  Vn+1 : Inport  Port=3
  T : Inport  Port=4  OutDataType=fixdt(1, 16)  OutScaling=2^0
  tau : Inport  Port=5  OutDataType=fixdt(1, 16)  OutScaling=2^0
  2·ab : Gain  Gain=2  ParameterDataType=fixdt(1, 16)  ParameterScaling=2^0  OutDataType=fixdt(1, 16)  OutScaling=2^0
  2·an : Gain  Gain=2  ParameterDataType=fixdt(1, 16)  ParameterScaling=2^0  OutDataType=fixdt(1, 16)  OutScaling=2^0
  Add1 : Sum  Inputs=+--  OutDataType=fixdt(1, 16)  OutScaling=2^-10
  Add2 : Sum  OutDataType=fixdt(1, 16)  OutScaling=2^-10
  Divide : Product  Inputs=/*  OutDataType=fixdt(1, 16)  OutScaling=2^-10
  Divide1 : Product  Inputs=*/  OutDataType=fixdt(1, 16)  OutScaling=2^-10
  Divide2 : Product  Inputs=/*  OutDataType=fixdt(1, 16)  OutScaling=2^-10
  Divide3 : Product  Inputs=*/  OutDataType=fixdt(1, 16)  OutScaling=2^-10
  Ln : Constant  Value=20  OutDataType=fixdt(1, 16)  OutScaling=2^0
  MinMax : MinMax  Inputs=2  OutDataType=fixdt(1, 16)  OutScaling=2^0
  Product : Product  OutDataType=fixdt(1, 16)  OutScaling=2^0  RndMeth=Zero
  Sf : Constant  Value=88  OutDataType=fixdt(1, 16)  OutScaling=2^0
  Subtract : Sum  Inputs=+-  OutDataType=fixdt(1, 16)  OutScaling=2^-10
  Sum : Sum  Inputs=|+-  OutDataType=fixdt(1, 16)  OutScaling=2^0
  Vn+1^2 : Math  Operator=magnitude^2  OutDataType=fixdt(1, 16)  OutScaling=2^0  SaturateOnIntegerOverflow=on
  Vn^2 : Math  Operator=magnitude^2  OutDataType=fixdt(1, 16)  OutScaling=2^0  SaturateOnIntegerOverflow=on
  Vn^2/2·an : Product  Inputs=*/  OutDataType=fixdt(1, 16)  OutScaling=2^-10
  ab : Constant  Value=1.7/0.3048  OutDataType=fixdt(1, 16)  OutScaling=2^0
  an : Constant  Value=3.4/0.3048  OutDataType=fixdt(1, 16)  OutScaling=2^0
  d* : Constant  Value=5  OutDataType=fixdt(1, 16)  OutScaling=2^0
  u : Outport
  wires:
  ab/1 -> 2·ab/1
  Vn^2/1 -> Vn^2/2·an/1
  2·an/1 -> Vn^2/2·an/2
  Vn+1^2/1 -> Divide1/1
  2·ab/1 -> Divide1/2
  Vn^2/2·an/1 -> Subtract/1
  Divide1/1 -> Subtract/2
  Subtract/1 -> Divide/2
  tau/1 -> Divide2/1, Divide/1, Product/2
  d*/1 -> Add1/2
  Ln/1 -> Add1/3
  Add1/1 -> Divide2/2
  Divide2/1 -> Add2/1
  Divide/1 -> Add2/2
  Xn-(Xn+1)/1 -> Add1/1
  Vn/1 -> Vn^2/1
  Vn+1/1 -> Vn+1^2/1, Sum/2
  an/1 -> 2·an/1
  Add2/1 -> MinMax/1
  Sf/1 -> MinMax/2
  MinMax/1 -> Sum/1
  Sum/1 -> Divide3/1
  Product/1 -> Divide3/2
  Divide3/1 -> u/1
  T/1 -> Product/1

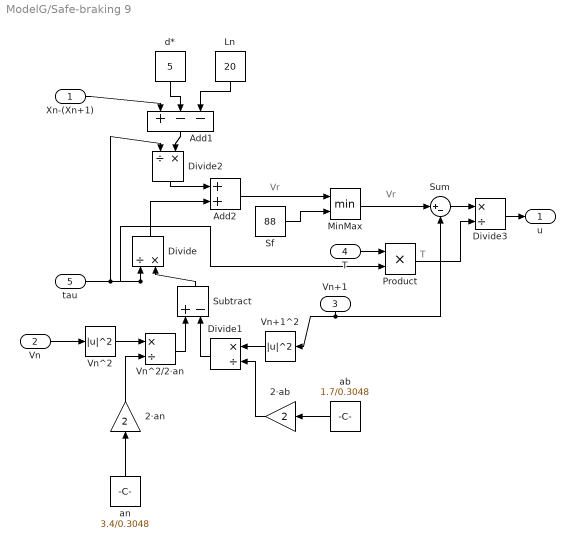
== system ModelG/Safe-braking 9 ==
  note: Vr
  note: Vr
  note: T
  Xn-(Xn+1) : Inport
  Vn : Inport  Port=2
  Vn+1 : Inport  Port=3
  T : Inport  Port=4  OutDataType=fixdt(1, 16)  OutScaling=2^0
  tau : Inport  Port=5  OutDataType=fixdt(1, 16)  OutScaling=2^0
  2·ab : Gain  Gain=2  ParameterDataType=fixdt(1, 16)  ParameterScaling=2^0  OutDataType=fixdt(1, 16)  OutScaling=2^0
  2·an : Gain  Gain=2  ParameterDataType=fixdt(1, 16)  ParameterScaling=2^0  OutDataType=fixdt(1, 16)  OutScaling=2^0
  Add1 : Sum  Inputs=+--  OutDataType=fixdt(1, 16)  OutScaling=2^-10
  Add2 : Sum  OutDataType=fixdt(1, 16)  OutScaling=2^-10
  Divide : Product  Inputs=/*  OutDataType=fixdt(1, 16)  OutScaling=2^-10
  Divide1 : Product  Inputs=*/  OutDataType=fixdt(1, 16)  OutScaling=2^-10
  Divide2 : Product  Inputs=/*  OutDataType=fixdt(1, 16)  OutScaling=2^-10
  Divide3 : Product  Inputs=*/  OutDataType=fixdt(1, 16)  OutScaling=2^-10
  Ln : Constant  Value=20  OutDataType=fixdt(1, 16)  OutScaling=2^0
  MinMax : MinMax  Inputs=2  OutDataType=fixdt(1, 16)  OutScaling=2^0
  Product : Product  OutDataType=fixdt(1, 16)  OutScaling=2^0  RndMeth=Zero
  Sf : Constant  Value=88  OutDataType=fixdt(1, 16)  OutScaling=2^0
  Subtract : Sum  Inputs=+-  OutDataType=fixdt(1, 16)  OutScaling=2^-10
  Sum : Sum  Inputs=|+-  OutDataType=fixdt(1, 16)  OutScaling=2^0
  Vn+1^2 : Math  Operator=magnitude^2  OutDataType=fixdt(1, 16)  OutScaling=2^0  SaturateOnIntegerOverflow=on
  Vn^2 : Math  Operator=magnitude^2  OutDataType=fixdt(1, 16)  OutScaling=2^0  SaturateOnIntegerOverflow=on
  Vn^2/2·an : Product  Inputs=*/  OutDataType=fixdt(1, 16)  OutScaling=2^-10
  ab : Constant  Value=1.7/0.3048  OutDataType=fixdt(1, 16)  OutScaling=2^0
  an : Constant  Value=3.4/0.3048  OutDataType=fixdt(1, 16)  OutScaling=2^0
  d* : Constant  Value=5  OutDataType=fixdt(1, 16)  OutScaling=2^0
  u : Outport
  wires:
  ab/1 -> 2·ab/1
  Vn^2/1 -> Vn^2/2·an/1
  2·an/1 -> Vn^2/2·an/2
  Vn+1^2/1 -> Divide1/1
  2·ab/1 -> Divide1/2
  Vn^2/2·an/1 -> Subtract/1
  Divide1/1 -> Subtract/2
  Subtract/1 -> Divide/2
  tau/1 -> Divide2/1, Divide/1, Product/2
  d*/1 -> Add1/2
  Ln/1 -> Add1/3
  Add1/1 -> Divide2/2
  Divide2/1 -> Add2/1
  Divide/1 -> Add2/2
  Xn-(Xn+1)/1 -> Add1/1
  Vn/1 -> Vn^2/1
  Vn+1/1 -> Vn+1^2/1, Sum/2
  an/1 -> 2·an/1
  Add2/1 -> MinMax/1
  Sf/1 -> MinMax/2
  MinMax/1 -> Sum/1
  Sum/1 -> Divide3/1
  Product/1 -> Divide3/2
  Divide3/1 -> u/1
  T/1 -> Product/1
